simulink model "FUZZY_Converter"  (R2023b)
settings: Solver=ode23tb  StartTime=0.0  StopTime=6  MaxStep=1e-4  RelTol=1e-4  EnableMultiTasking=on
undefined symbols (not defined in the file or in its folder): DiscIntNeverNeededParam, Ion, Lithium
libraries: spsDiodeLib x3, simulink x2, spsSeriesRLCBranchLib x2, fuzblock x2, spsBatteryLib x1, spsIdealSwitchLib x1, spsLinearTransformerLib x1, eePwmGenerator x1, spsDCVoltageSourceLib x1, spsVoltageMeasurementLib x1, sps_lib x1
settings Model: SimulationMode=accelerator  Creator=The MathWorks, Inc.  LastModifiedBy=User
settings SolverCC: AlgebraicLoopSolver=TrustRegion  SolverResetMethod=Robust
settings OptimizationCC: LifeSpan=inf
settings DebuggingCC: ReadBeforeWriteMsg=DisableAll  WriteAfterWriteMsg=DisableAll  WriteAfterReadMsg=DisableAll  MultiTaskDSMMsg=none  UnconnectedInputMsg=warning  UnconnectedOutputMsg=warning  UnconnectedLineMsg=warning  SFUnexpectedBacktrackingDiag=warning  SFNoUnconditionalDefaultTransitionDiag=warning  SFExecutionAtInitializationDiag=none  ArithmeticOperatorsInVariantConditions=warning
settings ModelReferenceCC: UpdateModelReferenceTargets=IfOutOfDate  EnableRefExpFcnMdlSchedulingChecks=on
settings SFSimCC: SFSimEcho=off  SimUseLocalCustomCode=off  CustomCodeUndefinedFunction=UseInterfaceOnly
settings RTWCC: RTWUseLocalCustomCode=off
settings CodeAppCC: StateflowObjectComments=on
settings GRTTargetCC: TargetLangStandard=C89/C90 (ANSI)
settings ConfigComp: CovMetricSettings=dw  CovSaveCumulativeToWorkspaceVar=on  CovSaveSingleToWorkspaceVar=on  CovExternalEMLEnable=off
settings SimscapeCC: SimscapeNormalizeSystem=off  SimscapeNominalValues={1, 'bar'; 1, 'cm^3/s'; 1, 'bar*kg/s'; 1, 'kJ/kg'; 1, 'kW'; }

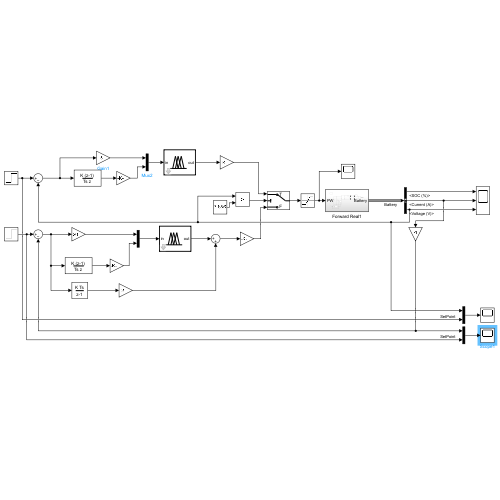
[thumbnail: Simulink's stored preview of the top-level diagram]
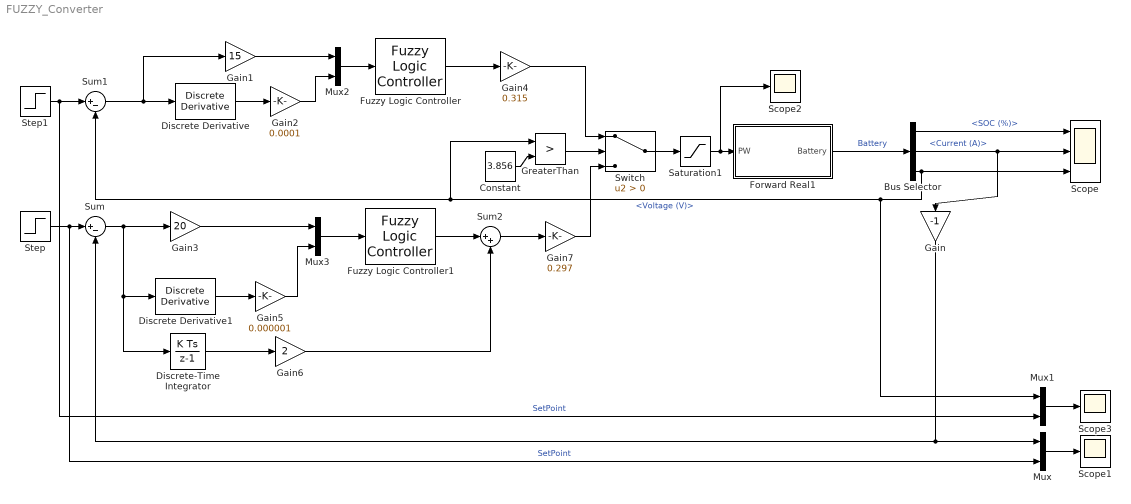
== system FUZZY_Converter ==
  Bus Selector : BusSelector  OutputSignals=SOC (%),Current (A),Voltage (V)
  Constant : Constant  Value=3.856  VectorParams1D=off
  Discrete Derivative : simulink/Discrete/Discrete Derivative  gainval=1.0  ICPrevScaledInput=0.0  OutMin=[]  OutMax=[]  OutDataType=fixdt(1, 16)  OutScaling=2^-10  DoSatur=off
  Discrete Derivative1 : simulink/Discrete/Discrete Derivative  gainval=1.0  ICPrevScaledInput=0.0  OutMin=[]  OutMax=[]  OutDataType=fixdt(1, 16)  OutScaling=2^-10  DoSatur=off
  Discrete-Time Integrator : DiscreteIntegrator  SampleTime=-1  ICPrevOutput=DiscIntNeverNeededParam  ICPrevScaledInput=DiscIntNeverNeededParam
  Forward Real1 : Subsystem
  Fuzzy Logic Controller : fuzblock/Fuzzy Logic  Controller  FIS='fisPD.fis'  OutputSampleNumber=101  DataType=double  FuzzifiedInputs=off  RuleFiringStrengths=off  RuleOutputs=off  AggregatedOutputs=off  SimulateUsing=Interpreted execution  OutOfRangeInputValueMessage=warning  NoRuleFiredMessage=warning  EmptyOutputFuzzySetMessage=warning
  Fuzzy Logic Controller1 : fuzblock/Fuzzy Logic  Controller  FIS='fisPD.fis'  OutputSampleNumber=101  DataType=double  FuzzifiedInputs=off  RuleFiringStrengths=off  RuleOutputs=off  AggregatedOutputs=off  SimulateUsing=Interpreted execution  OutOfRangeInputValueMessage=warning  NoRuleFiredMessage=warning  EmptyOutputFuzzySetMessage=warning
  Gain : Gain  Gain=-1
  Gain1 : Gain  Gain=15
  Gain2 : Gain  Gain=0.0001
  Gain3 : Gain  Gain=20
  Gain4 : Gain  Gain=0.315
  Gain5 : Gain  Gain=0.000001
  Gain6 : Gain  Gain=2
  Gain7 : Gain  Gain=0.297
  GreaterThan : RelationalOperator  Operator=>  OutDataTypeStr=boolean  ZeroCross=off  RndMeth=Simplest  InputSameDT=off
  Mux{,1..3} (4 alike) : Mux  Inputs=2
  Saturation1 : Saturate  UpperLimit=24  LowerLimit=0
  Scope : Scope  NumInputPorts=3
  Scope1 : Scope
  Scope2 : Scope
  Scope3 : Scope
  Step : Step  Time=0  After=0.3  SampleTime=0
  Step1 : Step  Time=0  After=3.856  SampleTime=0
  Sum : Sum  Inputs=|+-
  Sum1 : Sum  Inputs=|+-
  Sum2 : Sum  Inputs=|++
  Switch : Switch  Criteria=u2 > Threshold  SaturateOnIntegerOverflow=off  InputSameDT=off
  wires:
  Forward Real1/1(Battery) -> Bus Selector/1  "Battery"
  Bus Selector/3 -> Scope/3, Mux1/1, GreaterThan/1, Sum1/2  "<Voltage (V)>"
  Step/1 -> Mux/2, Sum/1  "SetPoint"
  Mux/1 -> Scope1/1
  Step1/1 -> Sum1/1, Mux1/2  "SetPoint"
  Mux1/1 -> Scope3/1
  Switch/1 -> Saturation1/1
  Saturation1/1 -> Forward Real1/1(PW), Scope2/1
  Constant/1 -> GreaterThan/2
  GreaterThan/1 -> Switch/2
  Gain/1 -> Mux/1, Sum/2
  Bus Selector/1 -> Scope/1  "<SOC (%)>"
  Bus Selector/2 -> Scope/2, Gain/1  "<Current (A)>"
  Gain2/1 -> Mux2/2
  Discrete Derivative/1 -> Gain2/1
  Mux2/1 -> Fuzzy Logic Controller/1
  Fuzzy Logic Controller/1 -> Gain4/1
  Gain1/1 -> Mux2/1
  Sum1/1 -> Gain1/1, Discrete Derivative/1
  Gain4/1 -> Switch/1
  Sum2/1 -> Gain7/1
  Fuzzy Logic Controller1/1 -> Sum2/1
  Gain3/1 -> Mux3/1
  Mux3/1 -> Fuzzy Logic Controller1/1
  Gain6/1 -> Sum2/2
  Gain5/1 -> Mux3/2
  Discrete Derivative1/1 -> Gain5/1
  Discrete-Time Integrator/1 -> Gain6/1
  Gain7/1 -> Switch/3
  Sum/1 -> Discrete-Time Integrator/1, Discrete Derivative1/1, Gain3/1

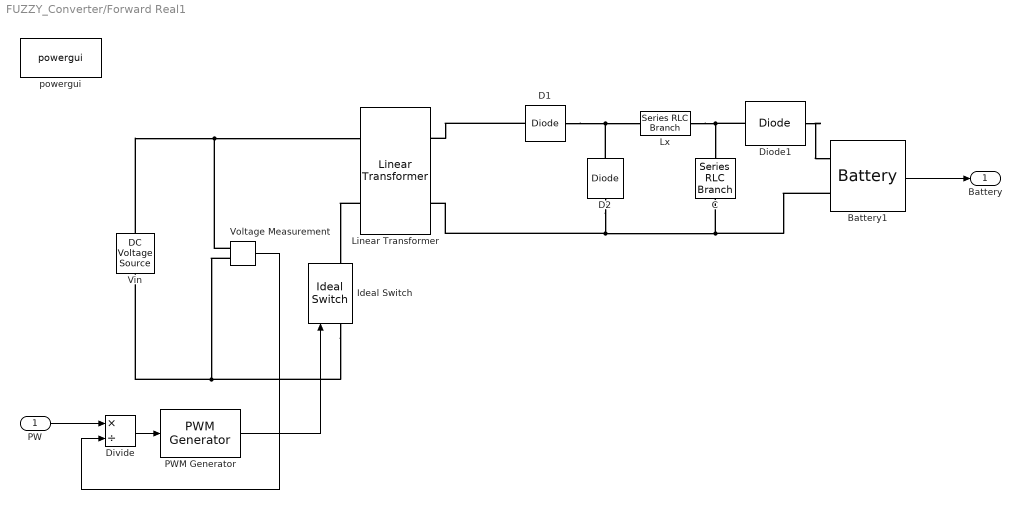
== system FUZZY_Converter/Forward Real1 ==
  PW : Inport
  Battery1 : spsBatteryLib/Battery  BatType=Lithium-Ion  ShowTempParam=off  ThermalPreset=no  ShowAgeParam=off  NomV=3.3  NomQ=1  SOC=99.8  Batt_Tr=30  PresetModel=on  MaxQ=1  MinV=2.475  FullV=3.8412  Dis_rate=0.43478  R=0.033  Normal_OP=0.90435  expZone="[3.5653     0.04913]"  current=[6.5 13 32.5]  Units=Time  Tci=20  NomT=20  T2=-30  MaxQ2=4.8  FullV2=7.1  Normal_OP2=5.655  expZone2="[6.58           1]"  Rca=0.6  ti=2000  Dp=0  Neq0=0  Tsim=1e6  Ta1=25  Qeol=5.4*0.9  Reol=0.013333*1.2  Char_age=[2.3478, 3]  Dis_age=[2.3478, 10]  N1=1500  N2=10500  N3=1000  N4=1400  Ta2=45  N5=950
  C : spsSeriesRLCBranchLib/Series RLC Branch  LConnTagsString=__new0  RConnTagsString=__new0  BranchType=C  Resistance=1e-4  Inductance=200e-6  SetiL0=off  InitialCurrent=0  Capacitance=10e-6  Setx0=off  InitialVoltage=0  Measurements=None
  D1 : spsDiodeLib/Diode  Ron=1e-3  Lon=0  Vf=0  IC=0  UseSnubber=off  Rs=inf  Cs=0  Measurements=off
  D2 : spsDiodeLib/Diode  Ron=1e-3  Lon=0  Vf=0  IC=0  UseSnubber=off  Rs=inf  Cs=0  Measurements=off
  Diode1 : spsDiodeLib/Diode  Ron=0  Lon=0  Vf=0  IC=0  UseSnubber=0  Rs=0  Cs=0  Measurements=off
  Divide : Product  Inputs=*/
  Ideal Switch : spsIdealSwitchLib/Ideal Switch  Ron=0.001  Lon=0  IC=0  Rs=1e5  Cs=inf  Measurements=on
  Linear Transformer : spsLinearTransformerLib/Linear Transformer  UNITS=SI  NominalPower=[ 25 100e3 ]  winding1=[48 0 0]  winding2=[48 0 0]  ThreeWindings=off  winding3=[48 0 0]  RmLm=[inf 10e-3]  Measurements=Magnetization current  DataType=on
  Lx : spsSeriesRLCBranchLib/Series RLC Branch  LConnTagsString=__new0  RConnTagsString=__new0  BranchType=L  Resistance=10  Inductance=1.33e-3  SetiL0=off  InitialCurrent=0  Capacitance=400e-6  Setx0=off  InitialVoltage=0  Measurements=Branch current
  PWM Generator : eePwmGenerator/PWM Generator  CarrCount=Down  Tper=0.0001  Tdelay=0  Ts=1e-6
  Vin : spsDCVoltageSourceLib/DC Voltage Source  Amplitude=24  Measurements=None
  Voltage Measurement : spsVoltageMeasurementLib/Voltage Measurement  PhasorSimulation=off  OutputType=Complex  PSBequivalent=0
  powergui : sps_lib/powergui  Priority=1  SimulationMode=Continuous  SampleTime=1e-6  frequency=60  Iterations=50  frequencyindice=0  Pbase=100e6  ErrMax=1e-4  UnitsV=kV  UnitsW=MW  buscounter=0  FunctionMessages=off  echomessages=off  EnableUseOfTLC=off  CurrentSourceSwitches=off  DisableSnubberDevices=off  DisableRonSwitches=off  DisableVfSwitches=off  DisplayEquations=off  AutomaticDiscreteSolvers=off  SolverType=Tustin/Backward Euler (TBE)  Interpol=off  ExternalGateDelay=off  methode=off  Ts=100  x0status=blocks  SPID=on  SwTol=0  HookPort=off  NonlinearTolerance=1e-4  nMaxIteration=100  ContinueOnMaxIteration=off  RestoreLinks=warning  ResistiveCurrentMeasurement=off  Frange=[0:2:500]  Ylog=off  Xlog=on  ShowGrid=off  save=off  variable=ZData  structure=0  ZoomFFT=off  StartTime=0.0  cycles=1  DisplayStyle=1  fundamental=60  FreqAxis=off  MaxFrequency=1000  frequencyindicesteady=1  RmsSteady=1  display=off
  Battery : Outport
  wires:
  PWM Generator/1 -> Ideal Switch/1
  Divide/1 -> PWM Generator/1
  PW/1 -> Divide/1
  Voltage Measurement/1 -> Divide/2
  Battery1/1 -> Battery/1
  connections:
  D2/LConn1 -- C/RConn1 -- Battery1/LConn2 -- Linear Transformer/RConn2
  Lx/RConn1 -- Diode1/LConn1 -- C/LConn1
  Vin/RConn1 -- Voltage Measurement/LConn1 -- Linear Transformer/LConn1
  Ideal Switch/LConn1 -- Voltage Measurement/LConn2 -- Vin/LConn1
  D2/RConn1 -- D1/RConn1 -- Lx/LConn1
  Linear Transformer/LConn2 -- Ideal Switch/RConn1
  D1/LConn1 -- Linear Transformer/RConn1
  Diode1/RConn1 -- Battery1/LConn1
